simulink model "untitled"  (R2021a)
settings: Solver=VariableStepAuto  StartTime=0.0  StopTime=10.0  RelTol=1e-3
settings Model: Creator=migue  LastModifiedBy=migue

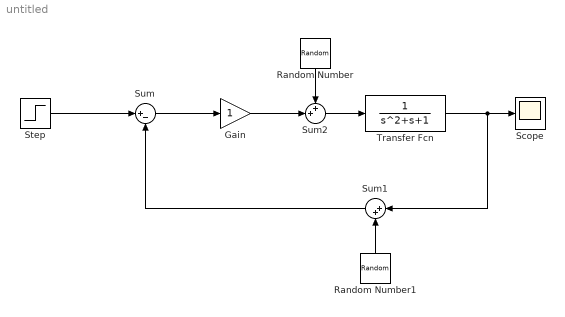
== system untitled ==
  Gain : Gain
  Random Number : RandomNumber  Variance=[0,0.1]  SampleTime=0.1
  Random Number1 : RandomNumber  Variance=[0,0.2]  SampleTime=0.1
  Scope : Scope
  Step : Step  After=2
  Sum : Sum  Inputs=|+-
  Sum1 : Sum  Inputs=|++
  Sum2 : Sum  Inputs=++|
  Transfer Fcn : TransferFcn  Denominator=[1 1 1]
  wires:
  Step/1 -> Sum/1
  Sum/1 -> Gain/1
  Sum1/1 -> Sum/2
  Transfer Fcn/1 -> Sum1/1, Scope/1
  Gain/1 -> Sum2/2
  Random Number/1 -> Sum2/1
  Random Number1/1 -> Sum1/2
  Sum2/1 -> Transfer Fcn/1
